simulink model "IV_2018B_test"  (R2018b)
settings: Solver=VariableStepAuto  StartTime=0.0  StopTime=105.0  RelTol=1e-3
libraries: fl_lib x23, nesl_utility x16, elec_lib x2
settings Model: Creator=94840  LastModifiedBy=WangMingcheng
settings DataIOCC: SaveFormat=Array

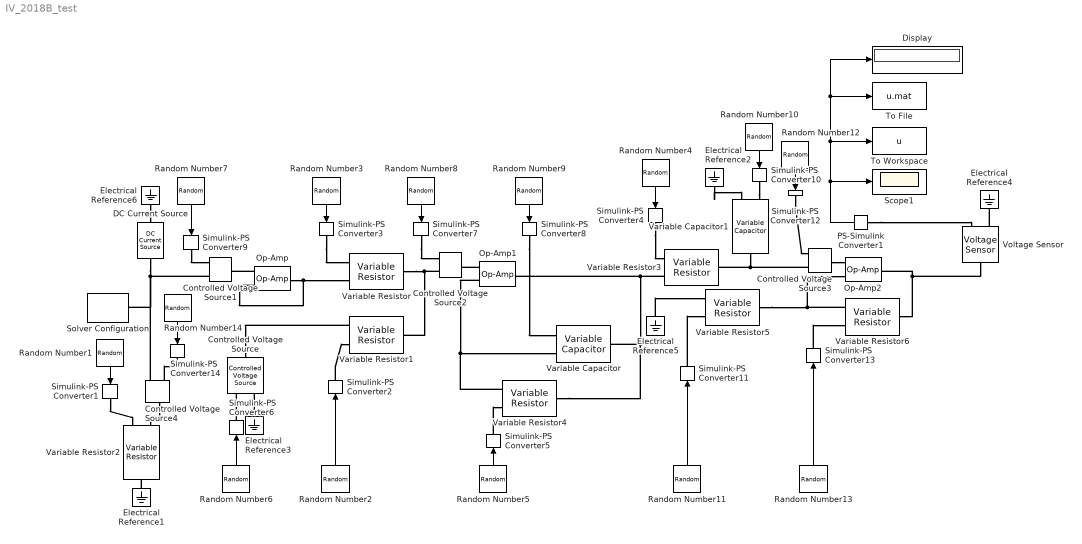
== system IV_2018B_test ==
  Controlled Voltage Source{,1..4} (5 alike) : fl_lib/Electrical/Electrical Sources/Controlled Voltage Source
  DC Current Source : fl_lib/Electrical/Electrical Sources/DC Current Source  i0=0.15 A
      settings: SourceProductName=Simscape  SourceProductBaseCode=SS
  Display : Display
  Electrical Reference{1..6} (6 alike) : fl_lib/Electrical/Electrical Elements/Electrical Reference
  Op-Amp : fl_lib/Electrical/Electrical Elements/Op-Amp  outI_specify=off  outI_priority=None  outI=0 A  outI_nominal_specify=off  outI_nominal_unit=A  outI_nominal_value=1
  Op-Amp1 : fl_lib/Electrical/Electrical Elements/Op-Amp  outI_specify=off  outI_priority=None  outI=0 A  outI_nominal_specify=off  outI_nominal_unit=A  outI_nominal_value=1
  Op-Amp2 : fl_lib/Electrical/Electrical Elements/Op-Amp  outI_specify=off  outI_priority=None  outI=0 A  outI_nominal_specify=off  outI_nominal_unit=A  outI_nominal_value=1
  PS-Simulink Converter1 : nesl_utility/PS-Simulink Converter  PhysicalDomain=network_engine_domain  SubClassName=ps_output  LeftPortType=input  RightPortType=output  PseudoPeriodic=off  Frequencies=[]  Unit=1  AffineConversion=off
  Random Number1 : RandomNumber  Mean=10  Variance=0.11111  Seed=698  SampleTime=0.001
  Random Number10 : RandomNumber  Mean=5e-5  Variance=0.0  Seed=843  SampleTime=0.001
  Random Number11 : RandomNumber  Mean=1000000  Variance=0.0  Seed=231  SampleTime=0.001
  Random Number12 : RandomNumber  Variance=0.0  Seed=256  SampleTime=0.001
  Random Number13 : RandomNumber  Mean=1  Variance=0.0  Seed=508  SampleTime=0.001
  Random Number14 : RandomNumber  Variance=0  SampleTime=0.001
  Random Number2 : RandomNumber  Mean=10000  Variance=0  Seed=711  SampleTime=0.001  VectorParams1D=off
  Random Number3 : RandomNumber  Mean=10000  Variance=0  Seed=980  SampleTime=0.001
  Random Number4 : RandomNumber  Mean=10000  Variance=0.0  Seed=395  SampleTime=0.001
  Random Number5 : RandomNumber  Mean=5100  Variance=0.0  Seed=162  SampleTime=0.001
  Random Number6 : RandomNumber  Mean=3.3  Variance=0.0  Seed=853  SampleTime=0.001
  Random Number7 : RandomNumber  Variance=0.0  Seed=320  SampleTime=0.001
  Random Number8 : RandomNumber  Variance=0.0  Seed=909  SampleTime=0.001
  Random Number9 : RandomNumber  Mean=1e-5  Variance=0.0  Seed=579  SampleTime=0.001  VectorParams1D=off
  Scope1 : Scope
  Simulink-PS Converter{1..14} (14 alike) : nesl_utility/Simulink-PS Converter  PhysicalDomain=network_engine_domain  SubClassName=ps_input  LeftPortType=input  RightPortType=output  PseudoPeriodic=off  Frequencies=[]  NoiseDistribution=none  NoiseParameters=[]  Unit=1  AffineConversion=off  FilteringAndDerivatives=provide  SimscapeFilterOrder=1  InputFilterTimeConstant=0.001  UdotUserProvided=0
  Solver Configuration : nesl_utility/Solver Configuration  PhysicalDomain=network_engine_domain  SubClassName=solver  LeftPortType=input  RightPortType=generic  Tones=[]  Harmonics=[]  SimulateNoise=off  Profile=off  UseLocalSampling=off  EnableSwitchedLinearOptims=on  FrequencyDomain=off  UseCCode=off  RelTol=0.001  AbsTol=1e-06  MinStep=1e-09  ToWorkspace=off  RevertToSquareIcSolve=off  NumHomotopyIterations=100  PhasorMode=off  PhasorModeNumHarmonics=1  DoDC=on  ResidualTolerance=1e-09  UseLocalSolver=on  LocalSolverChoice=NE_BACKWARD_EULER_ADVANCER  LocalSolverSampleTime=0.001  DoFixedCost=on  MaxNonlinIter=3  MaxModeIter=2  LinearAlgebra=auto  EquationFormulation=NE_TIME_EF  DelaysMemoryBudget=1024  AutomaticFiltering=on  FilteringTimeConstant=0.001  PartitionStorageMethod=AS_NEEDED  PartitionMemoryBudget=1024
  To File : ToFile  Filename=u.mat
  To Workspace : ToWorkspace  VariableName=u  SampleTime=-1
      settings: MaxDataPoints=100000  Save2DSignal=2-D array (concatenate along first dimension)
  Variable Capacitor : elec_lib/Passive Devices/Variable Capacitor  prm=2  Cmin=0.9 uF  r=1e-6 Ohm  v0=0 V  q0=0 C
      settings: SourceProductName=Simscape Electronics  SourceProductBaseCode=SN
  Variable Capacitor1 : elec_lib/Passive Devices/Variable Capacitor  prm=2  Cmin=45 uF  r=1e-6 Ohm  v0=0 V  q0=0 C
      settings: SourceProductName=Simscape Electronics  SourceProductBaseCode=SN
  Variable Resistor : fl_lib/Electrical/Electrical Elements/Variable Resistor  Rmin=9 kOhm  i_specify=off  i_priority=None  i=0 A  i_nominal_specify=off  i_nominal_unit=A  i_nominal_value=1  v_specify=off  v_priority=None  v=0 V  v_nominal_specify=off  v_nominal_unit=V  v_nominal_value=1
  Variable Resistor1 : fl_lib/Electrical/Electrical Elements/Variable Resistor  Rmin=9 kOhm  i_specify=off  i_priority=None  i=0 A  i_nominal_specify=off  i_nominal_unit=A  i_nominal_value=1  v_specify=off  v_priority=None  v=0 V  v_nominal_specify=off  v_nominal_unit=V  v_nominal_value=1
  Variable Resistor2 : fl_lib/Electrical/Electrical Elements/Variable Resistor  Rmin=9 Ohm  i_specify=off  i_priority=None  i=0 A  i_nominal_specify=off  i_nominal_unit=A  i_nominal_value=1  v_specify=off  v_priority=None  v=0 V  v_nominal_specify=off  v_nominal_unit=V  v_nominal_value=1
  Variable Resistor3 : fl_lib/Electrical/Electrical Elements/Variable Resistor  Rmin=9 kOhm  i_specify=off  i_priority=None  i=0 A  i_nominal_specify=off  i_nominal_unit=A  i_nominal_value=1  v_specify=off  v_priority=None  v=0 V  v_nominal_specify=off  v_nominal_unit=V  v_nominal_value=1
  Variable Resistor4 : fl_lib/Electrical/Electrical Elements/Variable Resistor  Rmin=4.5 kOhm  i_specify=off  i_priority=None  i=0 A  i_nominal_specify=off  i_nominal_unit=A  i_nominal_value=1  v_specify=off  v_priority=None  v=0 V  v_nominal_specify=off  v_nominal_unit=V  v_nominal_value=1
  Variable Resistor5 : fl_lib/Electrical/Electrical Elements/Variable Resistor  Rmin=0.9 MOhm  i_specify=off  i_priority=None  i=0 A  i_nominal_specify=off  i_nominal_unit=A  i_nominal_value=1  v_specify=off  v_priority=None  v=0 V  v_nominal_specify=off  v_nominal_unit=V  v_nominal_value=1
  Variable Resistor6 : fl_lib/Electrical/Electrical Elements/Variable Resistor  Rmin=0.9 Ohm  i_specify=off  i_priority=None  i=0 A  i_nominal_specify=off  i_nominal_unit=A  i_nominal_value=1  v_specify=off  v_priority=None  v=0 V  v_nominal_specify=off  v_nominal_unit=V  v_nominal_value=1
  Voltage Sensor : fl_lib/Electrical/Electrical Sensors/Voltage Sensor
  wires:
  Random Number1/1 -> Simulink-PS Converter1/1
  PS-Simulink Converter1/1 -> Display/1, To File/1, To Workspace/1, Scope1/1
  Random Number6/1 -> Simulink-PS Converter6/1
  Random Number7/1 -> Simulink-PS Converter9/1
  Random Number3/1 -> Simulink-PS Converter3/1
  Random Number2/1 -> Simulink-PS Converter2/1
  Random Number8/1 -> Simulink-PS Converter7/1
  Random Number5/1 -> Simulink-PS Converter5/1
  Random Number9/1 -> Simulink-PS Converter8/1
  Random Number4/1 -> Simulink-PS Converter4/1
  Random Number10/1 -> Simulink-PS Converter10/1
  Random Number11/1 -> Simulink-PS Converter11/1
  Random Number12/1 -> Simulink-PS Converter12/1
  Random Number13/1 -> Simulink-PS Converter13/1
  Random Number14/1 -> Simulink-PS Converter14/1
  connections:
  Controlled Voltage Source1/RConn2 -- Controlled Voltage Source4/RConn2 -- Solver Configuration/RConn1 -- DC Current Source/LConn1
  Simulink-PS Converter1/RConn1 -- Variable Resistor2/LConn1
  Simulink-PS Converter2/RConn1 -- Variable Resistor1/LConn1
  Electrical Reference1/LConn1 -- Variable Resistor2/RConn1
  Variable Resistor1/LConn2 -- Controlled Voltage Source/LConn1
  Electrical Reference3/LConn1 -- Controlled Voltage Source/RConn2
  Variable Resistor/RConn1 -- Controlled Voltage Source2/RConn2 -- Variable Resistor1/RConn1
  Variable Resistor3/LConn2 -- Op-Amp1/RConn1 -- Variable Resistor4/RConn1 -- Variable Capacitor/RConn1
  Voltage Sensor/RConn2 -- Electrical Reference4/LConn1
  PS-Simulink Converter1/LConn1 -- Voltage Sensor/RConn1
  Simulink-PS Converter4/RConn1 -- Variable Resistor3/LConn1
  Simulink-PS Converter5/RConn1 -- Variable Resistor4/LConn1
  Electrical Reference6/LConn1 -- DC Current Source/RConn1
  Op-Amp/RConn1 -- Variable Resistor/LConn2 -- Op-Amp/LConn2
  Simulink-PS Converter6/RConn1 -- Controlled Voltage Source/RConn1
  Variable Resistor4/LConn2 -- Op-Amp1/LConn2 -- Variable Capacitor/LConn2
  Op-Amp/LConn1 -- Controlled Voltage Source1/LConn1
  Simulink-PS Converter3/RConn1 -- Variable Resistor/LConn1
  Op-Amp1/LConn1 -- Controlled Voltage Source2/LConn1
  Simulink-PS Converter8/RConn1 -- Variable Capacitor/LConn1
  Variable Capacitor1/RConn1 -- Variable Resistor3/RConn1 -- Controlled Voltage Source3/RConn2
  Simulink-PS Converter10/RConn1 -- Variable Capacitor1/LConn1
  Electrical Reference2/LConn1 -- Variable Capacitor1/LConn2
  Simulink-PS Converter11/RConn1 -- Variable Resistor5/LConn1
  Variable Resistor5/RConn1 -- Variable Resistor6/LConn2 -- Op-Amp2/LConn2
  Electrical Reference5/LConn1 -- Variable Resistor5/LConn2
  Variable Resistor6/RConn1 -- Op-Amp2/RConn1 -- Voltage Sensor/LConn1
  Controlled Voltage Source3/LConn1 -- Op-Amp2/LConn1
  Simulink-PS Converter13/RConn1 -- Variable Resistor6/LConn1
  Controlled Voltage Source4/LConn1 -- Variable Resistor2/LConn2
  Simulink-PS Converter7/RConn1 -- Controlled Voltage Source2/RConn1
  Simulink-PS Converter9/RConn1 -- Controlled Voltage Source1/RConn1
  Controlled Voltage Source4/RConn1 -- Simulink-PS Converter14/RConn1
  Simulink-PS Converter12/RConn1 -- Controlled Voltage Source3/RConn1
